simulink model "sample_model7_coordinate_change_view_arrange"  (Simulink 7.0)
settings: Solver=ode45  StartTime=0.0  StopTime=10.0  RelTol=1e-3
PostLoadFcn:
  | View_ctr
InitFcn:
  | sample_file
values from neighbouring files (symbols this model uses):
  g = 9.81    [pid_parameters.m]    (also in sample_file.m)
  I = 0.0068    [pid_parameters.m]    (also in sample_file.m = 0.05)
  l = 0.4    [pid_parameters.m]    (also in sample_file.m = 0.3)
  m = 0.09    [pid_parameters.m]    (also in sample_file.m = 0.2)
  M = 0.6    [pid_parameters.m]    (also in sample_file.m = 0.5)
undefined symbols (not defined in the file or in its folder): rad, s
libraries: mblibv1 x10
settings Model: Creator=h-mita  LastModifiedBy=h-mita
settings DebuggingCC: SaveWithParameterizedLinksMsg=none

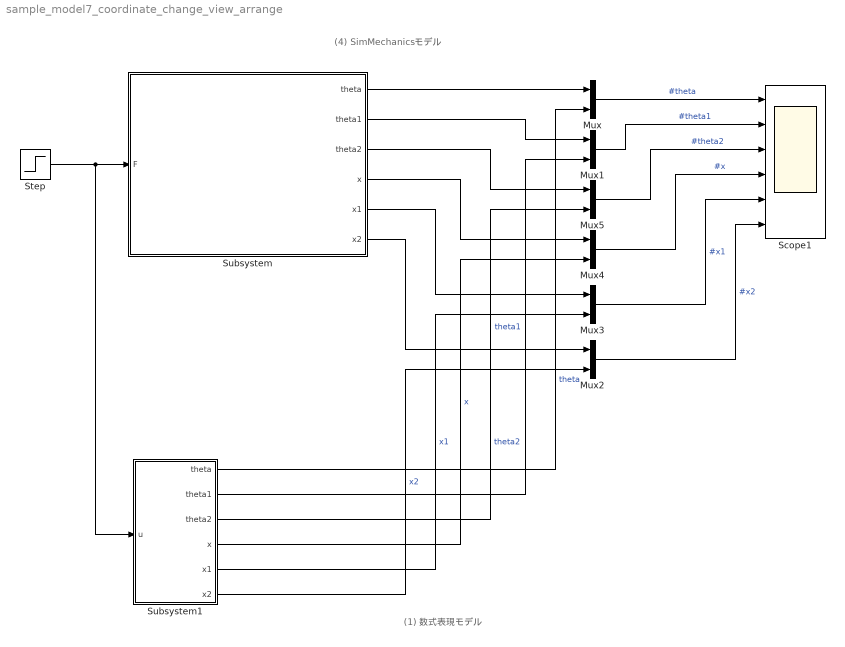
== system sample_model7_coordinate_change_view_arrange ==
  note: (1) 数式表現モデル
  note: (4) SimMechanicsモデル
  Mux{,1..5} (6 alike) : Mux  Inputs=2
  Scope1 : Scope  NumInputPorts=6
      settings: TimeRange=10  YMin=-10~-10~-50~0~-10~-20  YMax=20~10~50~60~20~20
  Step : Step  SampleTime=0
  Subsystem : Subsystem  mask{m=m, I=I, l=l, mass=M}
      mask prompts: m "m: 振子質量[kg]"; I "I: 振子慣性モーメント(y軸)[kgm^2]"; l "l: 振子重心までの長さ[m]"; mass "M: 台車質量[kg]"
      mask Display:
      | image(imread('千葉工大教科書.jpg'))
      | port_label('output',1,'theta')
      | port_label('output',2,'theta1')
      | port_label('output',3,'theta2')
      | port_label('output',4,'x')
      | port_label('output',5,'x1')
      | port_label('output',6,'x2')
  Subsystem1 : Subsystem
  wires:
  Step/1 -> Subsystem/1(F), Subsystem1/1(u)
  Subsystem/1(theta) -> Mux/1
  Subsystem1/1(theta) -> Mux/2  "theta"
  Subsystem/2(theta1) -> Mux1/1
  Subsystem1/2(theta1) -> Mux1/2  "theta1"
  Subsystem1/6(x2) -> Mux2/2  "x2"
  Subsystem/6(x2) -> Mux2/1
  Subsystem1/5(x1) -> Mux3/2  "x1"
  Subsystem/5(x1) -> Mux3/1
  Subsystem1/4(x) -> Mux4/2  "x"
  Subsystem/4(x) -> Mux4/1
  Subsystem1/3(theta2) -> Mux5/2  "theta2"
  Subsystem/3(theta2) -> Mux5/1
  Mux/1 -> Scope1/1  "#theta"
  Mux1/1 -> Scope1/2  "#theta1"
  Mux5/1 -> Scope1/3  "#theta2"
  Mux4/1 -> Scope1/4  "#x"
  Mux3/1 -> Scope1/5  "#x1"
  Mux2/1 -> Scope1/6  "#x2"

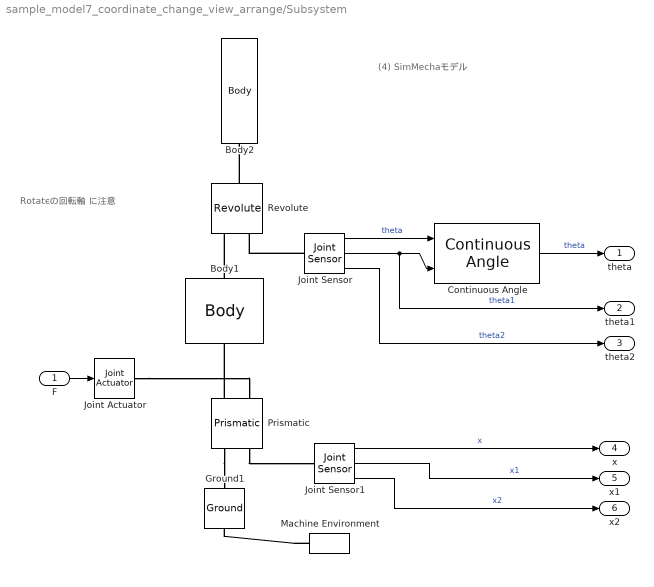
== system sample_model7_coordinate_change_view_arrange/Subsystem ==
  note: (4) SimMechaモデル
  note: Rotateの回転軸
      | に注意
  F : Inport
  Body1 : mblibv1/Bodies/Body  Tag=Factory generic  Description=Mechanical Blockset  Orientation=up  DialogController=MECH.DynMechDlgSource  PhysicalDomain=mechanical  SubClassName=Unknown  LeftPortType=workingframe  RightPortType=workingframe  LConnTagsString=CS1  RConnTagsString=CS2  DialogClass=MechanicalBodyBlock  Mass=mass  MassUnits=kg  InertiaUnits=kg*m^2  Inertia=eye(3)  Shape=Cylinder  ShapeDims=[1 1]  ShapeUnits=m  ShapeUse=false  Density=1  DensityUnits=kg/m^3  DensityUse=false  CG=Left$CG$[0 0 0]$WORLD$WORLD$m$[0 0 0]$Euler X-Y-Z$deg$WORLD$false  WorkingFrames=Left$CS1$[0 0 0]$WORLD$WORLD$m$[0 0 0]$Euler X-Y-Z$deg$WORLD$true#Right$CS2$[0 0 0]$WORLD$WORLD$m$[0 0 0]$Euler X-Y-Z$deg$WORLD$true  CGPos=[0 0 0]  CGRot=[0 0 0]  CS0Pos=[]  CS0Rot=[]  CS1Pos=[0 0 0]  CS1Rot=[0 0 0]  CS2Pos=[0 0 0]  CS2Rot=[0 0 0]  CS3Pos=[]  CS3Rot=[]  CS4Pos=[]  CS4Rot=[]  CS5Pos=[]  CS5Rot=[]  CS6Pos=[]  CS6Rot=[]  CS7Pos=[]  CS7Rot=[]  CS8Pos=[]  CS8Rot=[]  CS9Pos=[]  CS9Rot=[]  CS10Pos=[]  CS10Rot=[]  CS11Pos=[]  CS11Rot=[]  CS12Pos=[]  CS12Rot=[]  CS13Pos=[]  CS13Rot=[]  CS14Pos=[]  CS14Rot=[]  CS15Pos=[]  CS15Rot=[]  CS16Pos=[]  CS16Rot=[]  CS17Pos=[]  CS17Rot=[]  CS18Pos=[]  CS18Rot=[]  CS19Pos=[]  CS19Rot=[]  CS20Pos=[]  CS20Rot=[]
  Body2 : mblibv1/Bodies/Body  Tag=Factory generic  Description=Mechanical Blockset  Orientation=up  DialogController=MECH.DynMechDlgSource  PhysicalDomain=mechanical  SubClassName=Unknown  LeftPortType=workingframe  RightPortType=workingframe  LConnTagsString=CS1  RConnTagsString=CS2  DialogClass=MechanicalBodyBlock  Mass=m  MassUnits=kg  InertiaUnits=kg*m^2  Inertia=diag([0 I 0])  Shape=Cylinder  ShapeDims=[1 1]  ShapeUnits=m  ShapeUse=false  Density=1  DensityUnits=kg/m^3  DensityUse=false  CG=Left$CG$[0 0 l]$WORLD$WORLD$m$[0 0 0]$Euler X-Y-Z$deg$WORLD$false  WorkingFrames=Left$CS1$[0 0 0]$WORLD$WORLD$m$[0 0 0]$Euler X-Y-Z$deg$WORLD$true#Right$CS2$[0 0 l]$CG$CG$m$[0 0 0]$Euler X-Y-Z$deg$WORLD$true  CGPos=[0 0 l]  CGRot=[0 0 0]  CS0Pos=[]  CS0Rot=[]  CS1Pos=[0 0 0]  CS1Rot=[0 0 0]  CS2Pos=[0 0 l]  CS2Rot=[0 0 0]  CS3Pos=[]  CS3Rot=[]  CS4Pos=[]  CS4Rot=[]  CS5Pos=[]  CS5Rot=[]  CS6Pos=[]  CS6Rot=[]  CS7Pos=[]  CS7Rot=[]  CS8Pos=[]  CS8Rot=[]  CS9Pos=[]  CS9Rot=[]  CS10Pos=[]  CS10Rot=[]  CS11Pos=[]  CS11Rot=[]  CS12Pos=[]  CS12Rot=[]  CS13Pos=[]  CS13Rot=[]  CS14Pos=[]  CS14Rot=[]  CS15Pos=[]  CS15Rot=[]  CS16Pos=[]  CS16Rot=[]  CS17Pos=[]  CS17Rot=[]  CS18Pos=[]  CS18Rot=[]  CS19Pos=[]  CS19Rot=[]  CS20Pos=[]  CS20Rot=[]
  Continuous Angle : mblibv1/Utilities/Continuous Angle  SystemSampleTime=-1  rad=rad  rads=rad/s
  Ground1 : mblibv1/Bodies/Ground  Orientation=up  DialogController=MECH.DynMechDlgSource  SystemSampleTime=-1  LeftPortType=env  RightPortType=workingframe  PhysicalDomain=Mechanical  DialogClass=GroundBlock  CoordPosition=[0 0 0]  CoordPositionUnits=m  StateVectorMgrId=-1  MachineId=[0 0]  ShowEnvPort=on
  Joint Actuator : mblibv1/Sensors &  Actuators/Joint Actuator  Description=Mechanical Blockset  DialogController=MECH.DynMechDlgSource  SystemSampleTime=-1  PhysicalDomain=Mechanical  PortType=blob  ActuationStyle=Force  AngleUnits=deg  ArcVelocityUnits=deg/s  ArcAccelerationUnits=deg/s^2  CoordPositionUnits=m  VelocityUnits=m/s  AccelerationUnits=m/s^2  ForceUnits=N  TorqueUnits=N*m  ActiveIO=on  Width=1  DialogClass=MechanicalActuatorBlock  Primitive=P1  ReferenceFrame=Absolute (INERTIAL)
  Joint Sensor : mblibv1/Sensors &  Actuators/Joint Sensor  Description=Mechanical Blockset  DialogController=MECH.DynMechDlgSource  SystemSampleTime=-1  PhysicalDomain=Mechanical  PortType=blob  Muxed=off  Pose=off  Angle=on  AngleUnits=rad  ArcVelocity=on  ArcVelocityUnits=rad/s  ArcAcceleration=on  ArcAccelerationUnits=rad/s^2  CoordPosition=on  CoordPositionUnits=m  Velocity=off  VelocityUnits=m/s  Acceleration=off  AccelerationUnits=m/s^2  Quaternion=on  QuaternionDT=off  QuaternionDDT=off  QuaternionUnits=off  OutputVector=[ 1 ]  ActiveIO=on  Width=3  DialogClass=MechanicalSensorBlock  Primitive=R1  Force=off  ForceUnits=N  Torque=off  TorqueUnits=N*m  ReferenceFrame=Absolute (INERTIAL)  ReactionSensedSide=Base  ReactionReferenceFrame=Local (Body CS)  ReactionForce=off  ReactionForceUnits=N  ReactionMoment=off  ReactionMomentUnits=N*m
  Joint Sensor1 : mblibv1/Sensors &  Actuators/Joint Sensor  Description=Mechanical Blockset  DialogController=MECH.DynMechDlgSource  SystemSampleTime=-1  PhysicalDomain=Mechanical  PortType=blob  Muxed=off  Pose=off  Angle=on  AngleUnits=deg  ArcVelocity=off  ArcVelocityUnits=deg/s  ArcAcceleration=off  ArcAccelerationUnits=deg/s^2  CoordPosition=on  CoordPositionUnits=m  Velocity=on  VelocityUnits=m/s  Acceleration=on  AccelerationUnits=m/s^2  Quaternion=on  QuaternionDT=off  QuaternionDDT=off  QuaternionUnits=off  OutputVector=[ 1 ]  ActiveIO=on  Width=3  DialogClass=MechanicalSensorBlock  Primitive=P1  Force=off  ForceUnits=N  Torque=off  TorqueUnits=N*m  ReferenceFrame=Absolute (INERTIAL)  ReactionSensedSide=Base  ReactionReferenceFrame=Local (Body CS)  ReactionForce=off  ReactionForceUnits=N  ReactionMoment=off  ReactionMomentUnits=N*m
  Machine Environment : mblibv1/Bodies/Machine Environment  Tag=Factory ground  Orientation=left  DialogController=MECH.DialogSource  SystemSampleTime=-1  PortType=env  PhysicalDomain=Mechanical  DialogTemplateClass=MECH.MachineEnvironment  SyncWhenCopied=off  Gravity=[0 0 -9.81]  GravityUnits=m/s^2  GravityAsSignal=off  Dimensionality=Auto-detect  AnalysisType=Forward dynamics  LinearAssemblyTolerance=1e-3  LinearAssemblyToleranceUnits=m  AngularAssemblyTolerance=1e-3  AngularAssemblyToleranceUnits=rad  ConstraintSolverType=Stabilizing  ConstraintRelTolerance=1e-4  ConstraintAbsTolerance=1e-4  UseRobustSingularityHandling=off  RedundancyAnalysisToleranceType=Automatically select tolerance  RedundancyAnalysisTolerance=1e-14  StatePerturbationType=Fixed  PerturbationSize=1e-5  VisualizeMachine=off
  Prismatic : mblibv1/Joints/Prismatic  Tag=Factory generic  Description=Mechanical Blockset  Orientation=up  DialogController=MECH.DynMechDlgSource  PhysicalDomain=mechanical  SubClassName=Unknown  LeftPortType=blob  RightPortType=blob  LConnTagsString=__newl0|SA1  RConnTagsString=__newr0|SA1  NumSAPorts=2  CutJoint=off  MarkAsCut=off  Primitives=prismatic  PrimitiveProps=P1$World$[1 0 0]$prismatic  DialogClass=JointBlock  P1Axis=[1 0 0]
  Revolute : mblibv1/Joints/Revolute  Tag=Factory generic  Description=Mechanical Blockset  Orientation=up  DialogController=MECH.DynMechDlgSource  PhysicalDomain=mechanical  SubClassName=Unknown  LeftPortType=blob  RightPortType=blob  LConnTagsString=__newl0|SA1  RConnTagsString=__newr0  NumSAPorts=1  CutJoint=off  MarkAsCut=off  Primitives=revolute  PrimitiveProps=R1$World$[0 1 0]$revolute  DialogClass=JointBlock  R1Axis=[0 1 0]
  theta : Outport
  theta1 : Outport  Port=2
  theta2 : Outport  Port=3
  x : Outport  Port=4
  x1 : Outport  Port=5
  x2 : Outport  Port=6
  wires:
  Joint Sensor/1 -> Continuous Angle/1  "theta"
  Joint Sensor/2 -> Continuous Angle/2, theta1/1  "theta1"
  Continuous Angle/1 -> theta/1  "theta"
  Joint Sensor/3 -> theta2/1  "theta2"
  F/1 -> Joint Actuator/1
  Joint Sensor1/1 -> x/1  "x"
  Joint Sensor1/2 -> x1/1  "x1"
  Joint Sensor1/3 -> x2/1  "x2"
  connections:
  Prismatic/RConn1 -- Body1/LConn1
  Body1/RConn1 -- Revolute/LConn1
  Revolute/RConn1 -- Body2/LConn1
  Machine Environment/RConn1 -- Ground1/LConn1
  Prismatic/LConn1 -- Ground1/RConn1
  Joint Actuator/RConn1 -- Prismatic/RConn2
  Joint Sensor/LConn1 -- Revolute/LConn2
  Prismatic/LConn2 -- Joint Sensor1/LConn1

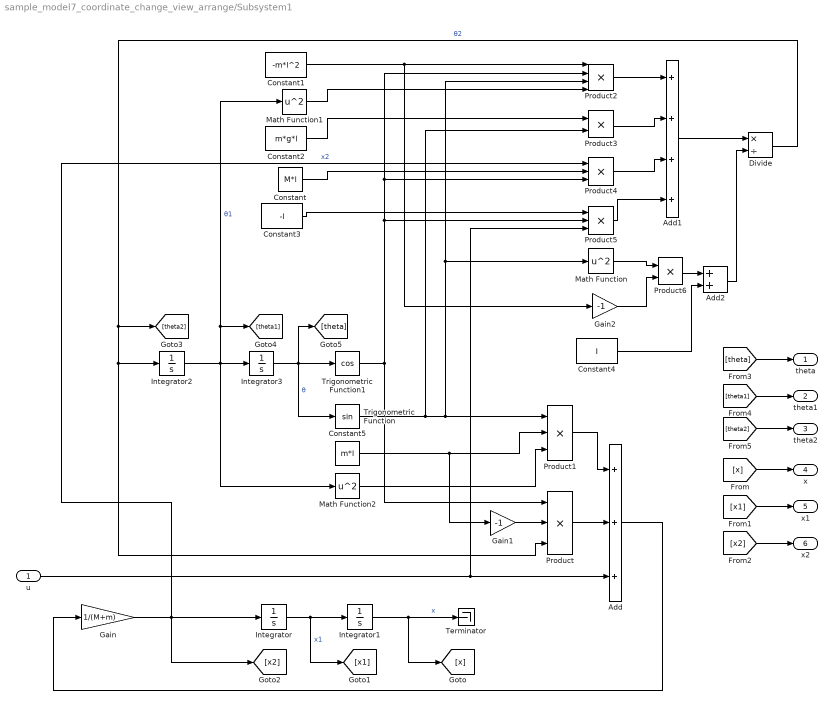
== system sample_model7_coordinate_change_view_arrange/Subsystem1 ==
  u : Inport  OutDataType=sfix(16)  OutScaling=2^0
  Add : Sum  Inputs=+++  OutDataType=sfix(16)  OutScaling=2^-10
  Add1 : Sum  Inputs=++++  OutDataType=sfix(16)  OutScaling=2^-10
  Add2 : Sum  OutDataType=sfix(16)  OutScaling=2^-10
  Constant : Constant  Value=M*l  OutDataType=sfix(16)  OutScaling=2^0
  Constant1 : Constant  Value=-m*l^2  OutDataType=sfix(16)  OutScaling=2^0
  Constant2 : Constant  Value=m*g*l  OutDataType=sfix(16)  OutScaling=2^0
  Constant3 : Constant  Value=-l  OutDataType=sfix(16)  OutScaling=2^0
  Constant4 : Constant  Value=I  OutDataType=sfix(16)  OutScaling=2^0
  Constant5 : Constant  Value=m*l  OutDataType=sfix(16)  OutScaling=2^0
  Divide : Product  Inputs=*/  OutDataType=sfix(16)  OutScaling=2^-10
  Gain : Gain  Gain=1/(M+m)  ParameterDataType=sfix(16)  ParameterScaling=2^0  OutDataType=sfix(16)  OutScaling=2^0
  Gain1 : Gain  Gain=-1  ParameterDataType=sfix(16)  ParameterScaling=2^0  OutDataType=sfix(16)  OutScaling=2^0
  Gain2 : Gain  Gain=-1  ParameterDataType=sfix(16)  ParameterScaling=2^0  OutDataType=sfix(16)  OutScaling=2^0
  Integrator{,1..3} (4 alike) : Integrator
  Math Function : Math  Operator=square  OutDataType=sfix(16)  OutScaling=2^0  SaturateOnIntegerOverflow=on
  Math Function1 : Math  Operator=square  OutDataType=sfix(16)  OutScaling=2^0  SaturateOnIntegerOverflow=on
  Math Function2 : Math  Operator=square  OutDataType=sfix(16)  OutScaling=2^0  SaturateOnIntegerOverflow=on
  Product{,1,4..5} (4 alike) : Product  Inputs=3  OutDataType=sfix(16)  OutScaling=2^0  RndMeth=Zero
  Product2 : Product  Inputs=4  OutDataType=sfix(16)  OutScaling=2^0  RndMeth=Zero
  Product3 : Product  OutDataType=sfix(16)  OutScaling=2^0  RndMeth=Zero
  Product6 : Product  OutDataType=sfix(16)  OutScaling=2^0  RndMeth=Zero
  Terminator : Terminator
  Trigonometric Function : Trigonometry
  Trigonometric Function1 : Trigonometry  Operator=cos
  theta : Outport  OutDataType=sfix(16)  OutScaling=2^0
  theta1 : Outport  Port=2  OutDataType=sfix(16)  OutScaling=2^0
  theta2 : Outport  Port=3  OutDataType=sfix(16)  OutScaling=2^0
  x : Outport  Port=4  OutDataType=sfix(16)  OutScaling=2^0
  x1 : Outport  Port=5  OutDataType=sfix(16)  OutScaling=2^0
  x2 : Outport  Port=6  OutDataType=sfix(16)  OutScaling=2^0
  wires:
  [x] -> x/1
  [x1] -> x1/1
  [x2] -> x2/1
  [theta] -> theta/1
  [theta1] -> theta1/1
  [theta2] -> theta2/1
  Integrator1/1 -> Terminator/1, [x]  "x"
  Add/1 -> Gain/1
  u/1 -> Product5/3, Add/3
  Add1/1 -> Divide/1
  Add2/1 -> Divide/2
  Constant4/1 -> Add2/2
  Product6/1 -> Add2/1
  Math Function/1 -> Product6/1
  Product5/1 -> Add1/4
  Product4/1 -> Add1/3
  Product3/1 -> Add1/2
  Product2/1 -> Add1/1
  Constant3/1 -> Product5/1
  Constant2/1 -> Product3/1
  Constant1/1 -> Product2/1, Gain2/1
  Product1/1 -> Add/1
  Trigonometric Function1/1 -> Product2/2, Product4/3, Product5/2, Product/1
  Product/1 -> Add/2
  Constant/1 -> Product4/2
  Trigonometric Function/1 -> Product3/2, Product2/3, Math Function/1, Product1/1
  Integrator3/1 -> Trigonometric Function/1, Trigonometric Function1/1, [theta]  "θ"
  Integrator2/1 -> [theta1], Math Function1/1, Integrator3/1, Math Function2/1  "θ1"
  Divide/1 -> Integrator2/1, Product/3, [theta2]  "θ2"
  Integrator/1 -> Integrator1/1, [x1]  "x1"
  Gain/1 -> Product4/1, Integrator/1, [x2]  "x2"
  Math Function1/1 -> Product2/4
  Gain2/1 -> Product6/2
  Gain1/1 -> Product/2
  Math Function2/1 -> Product1/3
  Constant5/1 -> Product1/2, Gain1/1
